simulink model "psbtransfo"  (Simulink 6.0)
settings: Solver=ode15s  SolverMode=SingleTasking  StartTime=0.0  StopTime=0.2  RelTol=1e-3  AbsTol=1e-6
libraries: powerlib2 x16, powerlib_extras x1
settings Model: Creator=patrice  LastModifiedBy=batserve  ExtModeTrigMode=oneshot  ExtModeArmWhenConnect=off  ExtModeAutoUpdateStatusClock=off
settings DataIOCC: LimitDataPoints=off  SignalLoggingName=sigsOut
settings OptimizationCC: BlockReduction=off  BooleanDataType=off
settings DebuggingCC: CheckExecutionContextPreStartOutputMsg=on  CheckExecutionContextRuntimeOutputMsg=on  SolverPrmCheckMsg=none
settings HardwareCC: TargetUnknown=on
settings RTWCC: TemplateMakefile=grt_unix.tmf

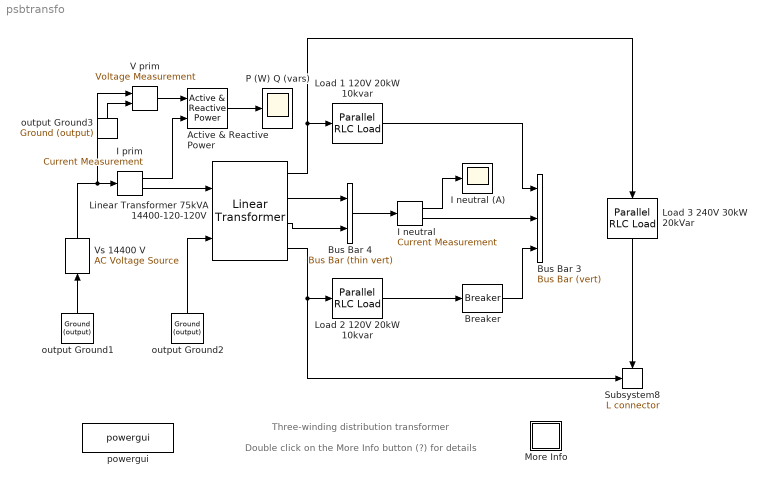
== system psbtransfo ==
  note: Three-winding distribution transformer
  note: Double click on the More Info button (?) for details
  Active & Reactive Power : powerlib_extras/Measurements/Active & Reactive Power  f1=60
  Breaker : powerlib2/Elements/Breaker  Tag=PoWeRsYsTeMbLoCk  a=1e-5  c=1  rs=inf  cs=0  times=[ .05 ]  Ts=0  comext=off  mesure=None  PSBOutputType=1
  Bus Bar 3 : powerlib2/Connectors/Bus Bar (vert)  Tag=PoWeRsYsTeMbLoCk  entrees=3  sorties=0  PSBOutputType=11111111111111111111111111111111111111111111111111111111111111111111111111111111111111111
  Bus Bar 4 : powerlib2/Connectors/Bus Bar (thin vert)  Tag=PoWeRsYsTeMbLoCk  input=2  output=1  PSBOutputType=111111111111111111111111111111111111111111111111111111111111111111111111111111111111
  I neutral : powerlib2/Measurements/Current Measurement  Tag=PoWeRsYsTeMmEaSuReMeNt  PhasorSimulation=off  OutputType=Magnitude  PSBOutputType=01  PSBequivalent=0
  I neutral (A) : Scope
      settings: TickLabels=on  TimeRange=0.2  YMin=-300  YMax=300  DataFormat=Array
  I prim : powerlib2/Measurements/Current Measurement  Tag=PoWeRsYsTeMmEaSuReMeNt  PhasorSimulation=off  OutputType=Magnitude  PSBOutputType=01  PSBequivalent=0
  Linear Transformer 75kVA 14400-120-120V : powerlib2/Elements/Linear Transformer  Tag=PoWeRsYsTeMbLoCk  a=[75e3,60]  b=[14.4e3 0.01,0.03]  c=[120,0.02,0]  w3check=on  d=[120,0.02,0]  e=[50,50]  mesure=None  PSBOutputType=1111
  Load 1 120V 20kW 10kvar : powerlib2/Elements/Parallel RLC Load  Tag=PoWeRsYsTeMbLoCk  a=120  b=60  c=20e3  d=10e3  e=0  mesure=None  PSBOutputType=1
  Load 2 120V 20kW 10kvar : powerlib2/Elements/Parallel RLC Load  Tag=PoWeRsYsTeMbLoCk  a=120  b=60  c=20e3  d=10e3  e=0  mesure=None  PSBOutputType=1
  Load 3 240V 30kW  20kVar : powerlib2/Elements/Parallel RLC Load  Tag=PoWeRsYsTeMbLoCk  Orientation=down  a=240  b=60  c=30e3  d=0  e=20e3  mesure=None  PSBOutputType=1
  More Info : Subsystem
      mask Display: disp('?')
  P (W) Q (vars) : Scope
      settings: TickLabels=on  TimeRange=0.2  YMin=-20000  YMax=80000  DataFormat=Array
  Subsystem8 : powerlib2/Connectors/L connector  Tag=PoWeRsYsTeMbLoCk
  V prim : powerlib2/Measurements/Voltage Measurement  Tag=PoWeRsYsTeMmEaSuReMeNt  PhasorSimulation=off  OutputType=Magnitude  PSBOutputType=0  PSBequivalent=0
  Vs 14400 V : powerlib2/Electrical Sources/AC Voltage Source  Tag=PoWeRsYsTeMbLoCk  Orientation=up  A=14400*sqrt(2)  P=0  F=60  stime=0  mesure=None  PSBOutputType=1
  output Ground1 : powerlib2/Connectors/Ground (output)  Tag=PoWeRsYsTeMbLoCk  Orientation=up  PSBOutputType=1
  output Ground2 : powerlib2/Connectors/Ground (output)  Tag=PoWeRsYsTeMbLoCk  Orientation=up  PSBOutputType=1
  output Ground3 : powerlib2/Connectors/Ground (output)  Tag=PoWeRsYsTeMbLoCk  Orientation=up  PSBOutputType=1
  powergui : powerlib2/powergui  Frange=logspace(0,3,50)  Ylog=off  Xlog=off  save=off  variable=ZData  ZoomFFT=on  StartTime=0.0  cycles=1  DisplayStyle=off  fundamental=60  FreqAxis=off  MaxFrequency=1000  frequencyindice=1  frequencyindicesteady=1  RmsSteady=1  display=off  Ts=0  methode=off  frequency=60  echomessages=off
  wires:
  output Ground1/1 -> Vs 14400 V/1
  I prim/2 -> Linear Transformer 75kVA 14400-120-120V/1
  output Ground2/1 -> Linear Transformer 75kVA 14400-120-120V/2
  Vs 14400 V/1 -> I prim/1, V prim/1
  I prim/1 -> Active & Reactive Power/2
  V prim/1 -> Active & Reactive Power/1
  Active & Reactive Power/1 -> P (W) Q (vars)/1
  output Ground3/1 -> V prim/2
  I neutral/2 -> Bus Bar 3/2
  I neutral/1 -> I neutral (A)/1
  Linear Transformer 75kVA 14400-120-120V/3 -> Bus Bar 4/2
  Linear Transformer 75kVA 14400-120-120V/2 -> Bus Bar 4/1
  Bus Bar 4/1 -> I neutral/1
  Linear Transformer 75kVA 14400-120-120V/1 -> Load 3 240V 30kW  20kVar/1, Load 1 120V 20kW 10kvar/1
  Load 1 120V 20kW 10kvar/1 -> Bus Bar 3/1
  Load 3 240V 30kW  20kVar/1 -> Subsystem8/Enable
  Linear Transformer 75kVA 14400-120-120V/4 -> Subsystem8/1, Load 2 120V 20kW 10kvar/1
  Load 2 120V 20kW 10kvar/1 -> Breaker/1
  Breaker/1 -> Bus Bar 3/3

== system psbtransfo/More Info ==
  note: This demonstration illustrates the  use of the linear transformer to simulate
      | a  three-winding distribution transformer rated 75 kVA - 14400/120/120 V.
  note: The transformer primary is connected to a high voltage source (14400 V rms).
      | Two identical inductive loads (20 kW -10 kvar) are connected to the two secondaries.
      | A third capacitive load (30 kW -20 kvar) is fed at 240 V.
      |
      | Initially, the circuit breaker in series with Load 2 is closed, so that the system is balanced.
  note: Open the powergui block to obtain the initial voltage and current phasors in steady state.
      | As loads are balanced the neutral current is practically  zero.
      |
      | Furthermore, as the inductive reactive power of Load 1 and Load 2 (2*10 kvar) is compensated by the capacitive reactive power
      | of Load 3 (20 kvar),the primary current is almost in phase with voltage  The small phase shift (-2.8deg.) is due to
      | the  reactive power associated with transformer reactive  losses.
      |
      | Open the two scopes and start the simulation. The following observations can be made:
      |
      | When the circuit breaker opens, a current starts to  flow in the neutral as a result of the load unbalance.
      | The active power computed from the primary voltage and current is measured by a Simulink block which can be found
      | in the "Extras/Measurement" library. When the breaker opens, the active power decreases from 70 kW to 50 kW.
  note: Circuit Description
  note: Demonstration
  note: G. Sybille (Hydro-Quebec)
